simulink subsystem "Day6_Scenario_1"  (R2024a)
settings: Solver=VariableStepAuto  StartTime=0.0  StopTime=10.0  RelTol=1e-3
libraries: CarMaker4SL x14
settings Model: Creator=junhyung.cha  LastModifiedBy=hajin

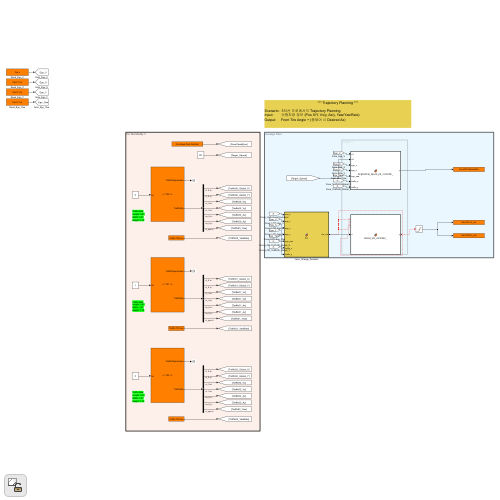
[thumbnail: Simulink's stored preview of the top-level diagram]
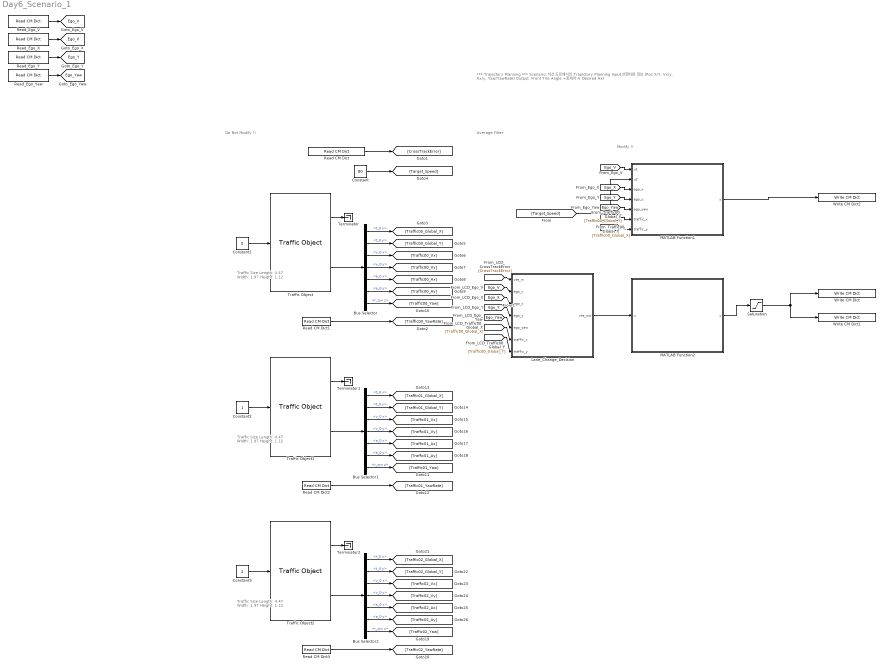
== system Day6_Scenario_1 ==
  note: Average Filter
  note: Do Not Modify !!
  note: Traffic Size
      | Length: 4.47
      | Width: 1.97
      | Height: 1.12
  note: Modify !!
  note: Traffic Size
      | Length: 4.47
      | Width: 1.97
      | Height: 1.12
  note: Traffic Size
      | Length: 4.47
      | Width: 1.97
      | Height: 1.12
  note: *** Trajectory Planning ***
      |
      | Scenario: 3차선 도로에서의 Trajectory Planning
      | Input: 선행차량 정보 (Pos X/Y, Vx/y, Ax/y, Yaw/YawRate)
      | Output: Front Tire Angle + (종제어 시 Desired Ax)
  Bus Selector : BusSelector  OutputSignals=t_0 x,t_0 y,v_0 x,v_0 y,a_0 x,a_0 y,r_zyx z
  Bus Selector1 : BusSelector  OutputSignals=t_0 x,t_0 y,v_0 x,v_0 y,a_0 x,a_0 y,r_zyx z
  Bus Selector2 : BusSelector  OutputSignals=t_0 x,t_0 y,v_0 x,v_0 y,a_0 x,a_0 y,r_zyx z
  Constant : Constant  Value=80
  Constant1 : Constant  Value=0
  Constant2 : Constant
  Constant3 : Constant  Value=2
  Lane_Change_Decision : MATLAB Function  TreatAsAtomicUnit=on
  MATLAB Function1 : MATLAB Function  TreatAsAtomicUnit=on
  MATLAB Function2 : MATLAB Function  TreatAsAtomicUnit=on
  Read CM Dict : CarMaker4SL/Read CM Dict  xname=Car.Road.Path.DevDist  xsync=off  xstime=Inherited
  Read CM Dict1 : CarMaker4SL/Read CM Dict  xname=Traffic.T00.rzv  xsync=off  xstime=Inherited
  Read CM Dict2 : CarMaker4SL/Read CM Dict  xname=Traffic.T01.rzv  xsync=off  xstime=Inherited
  Read CM Dict3 : CarMaker4SL/Read CM Dict  xname=Traffic.T02.rzv  xsync=off  xstime=Inherited
  Read_Ego_V : CarMaker4SL/Read CM Dict  xname=Car.v  xsync=off  xstime=Inherited
  Read_Ego_X : CarMaker4SL/Read CM Dict  xname=Car.Fr1.tx  xsync=off  xstime=Inherited
  Read_Ego_Y : CarMaker4SL/Read CM Dict  xname=Car.Fr1.ty  xsync=off  xstime=Inherited
  Read_Ego_Yaw : CarMaker4SL/Read CM Dict  xname=Car.Fr1.rz  xsync=off  xstime=Inherited
  Saturation : Saturate  UpperLimit=2  LowerLimit=-2
  Terminator : Terminator
  Terminator1 : Terminator
  Terminator2 : Terminator
  Traffic Object : CarMaker4SL/Traffic Object  xname=T00  ximode=Traffic Id  xstime=Inherited
      settings: SourceProductName=CarMaker4SL
  Traffic Object1 : CarMaker4SL/Traffic Object  xname=T01  ximode=Traffic Id  xstime=Inherited
      settings: SourceProductName=CarMaker4SL
  Traffic Object2 : CarMaker4SL/Traffic Object  xname=T02  ximode=Traffic Id  xstime=Inherited
      settings: SourceProductName=CarMaker4SL
  Write CM Dict : CarMaker4SL/Write CM Dict  xname=Car.CFL.rz_ext  xsync=off
  Write CM Dict1 : CarMaker4SL/Write CM Dict  xname=Car.CFR.rz_ext  xsync=off
  Write CM Dict2 : CarMaker4SL/Write CM Dict  xname=AccelCtrl.DesiredAx  xsync=off
  tag scope: Ego_V=global, Ego_X=global, Ego_Y=global, Ego_Yaw=global
  wires:
  Saturation/1 -> Write CM Dict1/1, Write CM Dict/1
  Constant1/1 -> Traffic Object/1
  MATLAB Function1/1(y) -> Write CM Dict2/1
  Read CM Dict/1 -> [CrossTrackError]
  [Target_Speed] -> MATLAB Function1/2(u2)
  Constant/1 -> [Target_Speed]
  Bus Selector/4 -> [Traffic00_Vy]  "<v_0 y>"
  Traffic Object/1 -> Terminator/1
  Bus Selector/3 -> [Traffic00_Vx]  "<v_0 x>"
  Traffic Object/2 -> Bus Selector/1
  Bus Selector/1 -> [Traffic00_Global_X]  "<t_0 x>"
  Bus Selector/2 -> [Traffic00_Global_Y]  "<t_0 y>"
  Read CM Dict1/1 -> [Traffic00_YawRate]
  Bus Selector/5 -> [Traffic00_Ax]  "<a_0 x>"
  Bus Selector/6 -> [Traffic00_Ay]  "<a_0 y>"
  Bus Selector/7 -> [Traffic00_Yaw]  "<r_zyx z>"
  Read CM Dict2/1 -> [Traffic01_YawRate]
  Bus Selector1/1 -> [Traffic01_Global_X]  "<t_0 x>"
  Bus Selector1/5 -> [Traffic01_Ax]  "<a_0 x>"
  Bus Selector1/6 -> [Traffic01_Ay]  "<a_0 y>"
  Bus Selector1/7 -> [Traffic01_Yaw]  "<r_zyx z>"
  Traffic Object1/1 -> Terminator1/1
  Bus Selector1/4 -> [Traffic01_Vy]  "<v_0 y>"
  Constant2/1 -> Traffic Object1/1
  Traffic Object1/2 -> Bus Selector1/1
  Bus Selector1/3 -> [Traffic01_Vx]  "<v_0 x>"
  Bus Selector1/2 -> [Traffic01_Global_Y]  "<t_0 y>"
  Bus Selector2/3 -> [Traffic02_Vx]  "<v_0 x>"
  Bus Selector2/2 -> [Traffic02_Global_Y]  "<t_0 y>"
  Traffic Object2/2 -> Bus Selector2/1
  Bus Selector2/1 -> [Traffic02_Global_X]  "<t_0 x>"
  Bus Selector2/6 -> [Traffic02_Ay]  "<a_0 y>"
  Constant3/1 -> Traffic Object2/1
  Traffic Object2/1 -> Terminator2/1
  Bus Selector2/7 -> [Traffic02_Yaw]  "<r_zyx z>"
  Bus Selector2/5 -> [Traffic02_Ax]  "<a_0 x>"
  Read CM Dict3/1 -> [Traffic02_YawRate]
  Bus Selector2/4 -> [Traffic02_Vy]  "<v_0 y>"
  Read_Ego_V/1 -> [Ego_V]
  Read_Ego_X/1 -> [Ego_X]
  Read_Ego_Y/1 -> [Ego_Y]
  Read_Ego_Yaw/1 -> [Ego_Yaw]
  [Ego_V] -> MATLAB Function1/1(u1)
  [Ego_X] -> MATLAB Function1/3(ego_x)
  [Ego_Y] -> MATLAB Function1/4(ego_y)
  [Ego_Yaw] -> MATLAB Function1/5(ego_yaw)
  [Traffic00_Global_X] -> MATLAB Function1/6(traffic_x)
  [Traffic00_Global_Y] -> MATLAB Function1/7(traffic_y)
  [CrossTrackError] -> Lane_Change_Decision/1(cte_in)
  [Ego_V] -> Lane_Change_Decision/2(ego_v)
  [Ego_X] -> Lane_Change_Decision/3(ego_x)
  [Ego_Y] -> Lane_Change_Decision/4(ego_y)
  [Ego_Yaw] -> Lane_Change_Decision/5(ego_yaw)
  [Traffic00_Global_X] -> Lane_Change_Decision/6(traffic_x)
  [Traffic00_Global_Y] -> Lane_Change_Decision/7(traffic_y)
  Lane_Change_Decision/1(cte_out) -> MATLAB Function2/1(u)
  MATLAB Function2/1(y) -> Saturation/1

== matlab function Day6_Scenario_1/Lane_Change_Decision ==
  data: cte_in input; ego_v input; ego_x input; ego_y input; ego_yaw input; traffic_x input; traffic_y input; cte_out output
function cte_out = fcn(cte_in, ego_v, ego_x, ego_y, ego_yaw, traffic_x, traffic_y)
%#codegen
% Lane Change Decision: 앞차 가까우면 좌측 차선 변경 → 추월 → 복귀
% State: 0=LK, 1=LC_OUT, 2=LC_PASS, 3=LC_BACK

persistent state t_in_state
if isempty(state)
    state = int32(0); t_in_state = 0;
end

TS = 0.001;

% ★ 차선 변경 offset 축소: 3.5 → 3.0
%   CarMaker 시나리오 실제 차선폭 < 3.5m일 가능성. 도로 이탈 방지
LANE_WIDTH = 3.0;

% ★ 더 천천히 부드럽게 변경: 3.0s → 4.0s
LC_TIME = 4.0;

PASS_DIST = -15.0;

% 트리거 거리: 속도 비례 (TTC ~3초)
TRIGGER_DIST = max(40.0, ego_v * 3.0);

% 자차 frame 종/횡 거리
dx = traffic_x - ego_x;
dy = traffic_y - ego_y;
long_dist = cos(ego_yaw)*dx + sin(ego_yaw)*dy;
lat_dist  = -sin(ego_yaw)*dx + cos(ego_yaw)*dy;

t_in_state = t_in_state + TS;

% State Machine
switch state
    case int32(0)  % LK
        if long_dist > 0.5 && long_dist < TRIGGER_DIST && abs(lat_dist) < 1.8 && ego_v > 5
            state = int32(1); t_in_state = 0;
        end

    case int32(1)  % LC_OUT
        if t_in_state >= LC_TIME
            state = int32(2); t_in_state = 0;
        end

    case int32(2)  % LC_PASS
        if long_dist < PASS_DIST || long_dist > 150
            state = int32(3); t_in_state = 0;
        end

    case int32(3)  % LC_BACK
        if t_in_state >= LC_TIME
            state = int32(0); t_in_state = 0;
        end
end

% Offset (smooth quintic ramp)
switch state
    case int32(0)
        target_offset = 0;
    case int32(1)
        s = min(1, t_in_state / LC_TIME);
        target_offset = -LANE_WIDTH * (10*s^3 - 15*s^4 + 6*s^5);
    case int32(2)
        target_offset = -LANE_WIDTH;
    case int32(3)
        s = min(1, t_in_state / LC_TIME);
        target_offset = -LANE_WIDTH * (1 - (10*s^3 - 15*s^4 + 6*s^5));
    otherwise
        target_offset = 0;
end

cte_out = cte_in - target_offset;
end

== matlab function Day6_Scenario_1/MATLAB Function1 ==
  settings: sampleTime=0.1
  data: u1 input; y output; u2 input; ego_x input; ego_y input; ego_yaw input; traffic_x input; traffic_y input
function y = longitudinal_speed_pd_controller_(u1, u2, ego_x, ego_y, ego_yaw, traffic_x, traffic_y)

% Longitudinal Controller: Speed PD + ACC + 같은 차선 필터
% u1: 자차 속도 [m/s] (Car.v)
% u2: 목표 속도 [km/h] (Target_Speed = 80)
% ego_x, ego_y, ego_yaw: 자차 글로벌 위치/방향
% traffic_x, traffic_y: 선행차 글로벌 위치
% y: 가속도 명령 [m/s^2]

persistent e_prev
if isempty(e_prev), e_prev = 0; end

% 1) 단위 통일
target_ms = u2 / 3.6;

% 2) 자차 frame 기준 종/횡 거리 계산
dx = traffic_x - ego_x;
dy = traffic_y - ego_y;
long_dist_raw = cos(ego_yaw) * dx + sin(ego_yaw) * dy;
lat_dist      = -sin(ego_yaw) * dx + cos(ego_yaw) * dy;

% 3) ★ 같은 차선 필터 (횡방향 1.8m 이내만 자차 차선)
LANE_HALF_WIDTH = 1.8;
if abs(lat_dist) > LANE_HALF_WIDTH
    % 옆 차선 차 → 무시
    long_dist = 1000;
else
    long_dist = long_dist_raw;
end

% 4) 안전 거리: 2초 시간갭 + 최소 10m
safe_dist = 10 + 2.0 * u1;

% 5) 속도 오차
e_v = target_ms - u1;

% 6) 거리 오차
if long_dist > 0.5 && long_dist < 150
    e_d = long_dist - safe_dist;
else
    e_d = 1000;
end

% 7) ACC: 거리/속도 중 더 보수적 선택
if e_d < e_v
    e_eff = e_d;
else
    e_eff = e_v;
end

% 8) PD 제어
de = e_eff - e_prev;
e_prev = e_eff;
Kp = 0.8; Kd = 0.1;
y = Kp * e_eff + Kd * de;

% 9) 비상 제동
if long_dist > 0.5 && long_dist < 5
    y = -6;
end
if y >  3, y =  3; end
if y < -6, y = -6; end

end

== matlab function Day6_Scenario_1/MATLAB Function2 ==
  settings: sampleTime=0.1
  data: u input; y output
function y = lateral_pid_controller_(u)

% Lateral PID — Cross-Track Error 보정 (순수 PID)
% u : modified_CTE (Lane_Change_Decision 출력)
% y : 앞바퀴 조향각 [rad]

persistent e_prev e_int
if isempty(e_prev)
    e_prev = 0; e_int = 0;
end

e  = -u;
de = e - e_prev;
e_int = e_int + e * 0.001;
e_prev = e;

% Anti-windup ±3.0
if e_int >  3.0,  e_int =  3.0; end
if e_int < -3.0,  e_int = -3.0; end

% 강화된 PID 게인
Kp = 1.5;
Ki = 0.3;
Kd = 0.4;

y = Kp * e + Ki * e_int + Kd * de;

% 조향각 한계 ±30°
if y >  pi/6, y =  pi/6; end
if y < -pi/6, y = -pi/6; end

end
